simulink model "chap1_3"  (R2016a)
settings: Solver=VariableStepAuto  StartTime=0.0  StopTime=10.0  RelTol=1e-3
settings Model: Creator=admin  LastModifiedBy=admin

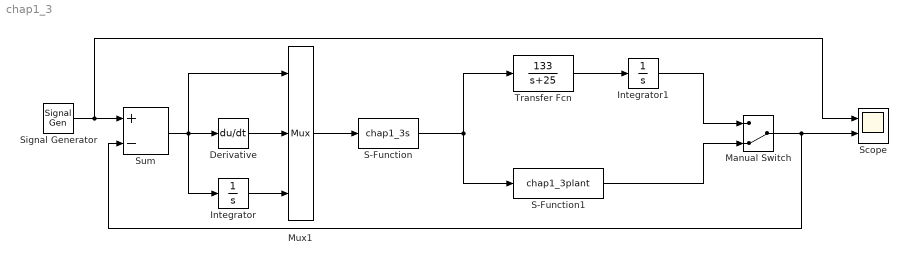
== system chap1_3 ==
  Derivative : Derivative
  Integrator : Integrator
  Integrator1 : Integrator
  Manual Switch : ManualSwitch  CurrentSetting=0
  Mux1 : Mux  Inputs=3
  S-Function : S-Function  FunctionName=chap1_3s  SFunctionDeploymentMode=off  EnableBusSupport=off
  S-Function1 : S-Function  FunctionName=chap1_3plant  SFunctionDeploymentMode=off  EnableBusSupport=off
  Scope : Scope  NumInputPorts=2
  Signal Generator : SignalGenerator  Frequency=0.2
  Sum : Sum  Inputs=+-
  Transfer Fcn : TransferFcn  Numerator=[133]  Denominator=[1 25]
  wires:
  Signal Generator/1 -> Scope/1, Sum/1
  S-Function/1 -> S-Function1/1, Transfer Fcn/1
  S-Function1/1 -> Manual Switch/2
  Manual Switch/1 -> Scope/2, Sum/2
  Sum/1 -> Mux1/1, Integrator/1, Derivative/1
  Integrator/1 -> Mux1/3
  Derivative/1 -> Mux1/2
  Mux1/1 -> S-Function/1
  Transfer Fcn/1 -> Integrator1/1
  Integrator1/1 -> Manual Switch/1
